simulink model "Cubesat_Control_PD"  (R2025b)
settings: Solver=ode45  StartTime=0.0  StopTime=t_stop  RelTol=1e-3
values from neighbouring files (symbols this model uses):
  J = 0.000634    [Matlab_to_BLE2.m]    (also in Run_CubeSat_HIL.m; init_simulation_lqr.m; init_simulation_pd.m)
  Jw = 4.607e-5    (= 4.607e-05)    [Matlab_to_BLE2.m]    (also in Run_CubeSat_HIL.m; init_simulation_lqr.m; init_simulation_pd.m)
  Kd = J * (3 * lambda - tau_delay)    [Matlab_to_BLE2.m]    (also in Run_CubeSat_HIL.m = 0.01; init_simulation_pd.m = J * (3 * lambda - tau))
  Kd_detumble = 0.03    [Matlab_to_BLE2.m]    (also in Run_CubeSat_HIL.m; init_simulation_lqr.m = lqr(A_d, B_d, Q_d, R_d); init_simulation_pd.m = 0.003)
  Ki = J * (lambda^3)    [Matlab_to_BLE2.m]    (also in init_simulation_pd.m)
  Kp = 3 * J * (lambda^2)    [Matlab_to_BLE2.m]    (also in Run_CubeSat_HIL.m = 0.02; init_simulation_pd.m)
  omega0 = deg2rad(omega0_deg)    [init_simulation_lqr.m]    (also in init_simulation_pd.m)
  omega_th_high = deg2rad(10)    [Run_CubeSat_HIL.m]    (also in init_simulation_lqr.m = deg2rad(10000); init_simulation_pd.m = deg2rad(10000))
  omega_th_low = deg2rad(2.0)    [Run_CubeSat_HIL.m]    (also in init_simulation_lqr.m = deg2rad(0.3); init_simulation_pd.m = deg2rad(0.3))
  omega_w0 = 0    [init_simulation_lqr.m]    (also in init_simulation_pd.m)
  tau = history_tau    [analyze_multiple_experiments.m]    (also in init_simulation_lqr.m = 2.3; init_simulation_pd.m = 2.3)
  tau_max = 0.2    [Matlab_to_BLE2.m]    (also in Run_CubeSat_HIL.m = 0.002; analyze_multiple_experiments.m = 0.002; init_simulation_lqr.m = 0.002; init_simulation_pd.m = 0.002)
  theta0 = theta(1)    [analyze_multiple_experiments.m]    (also in init_simulation_lqr.m = deg2rad(0); init_simulation_pd.m = deg2rad(0))
  theta_ref = deg2rad(theta_ref_deg)    [Matlab_to_BLE2.m]    (also in analyze_multiple_experiments.m = theta_ref_deg; init_simulation_lqr.m; init_simulation_pd.m)
settings Model: Creator=bbtp  LastModifiedBy=bbtp

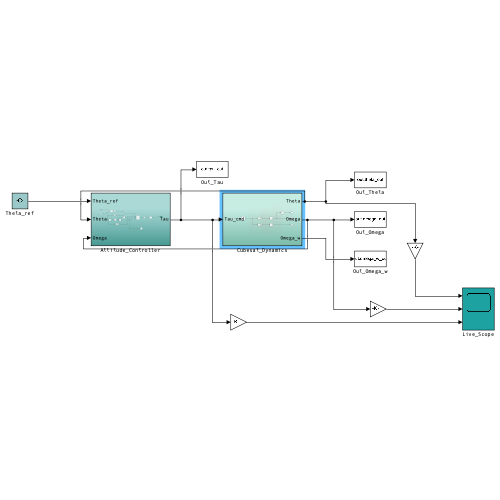
[thumbnail: Simulink's stored preview of the top-level diagram]
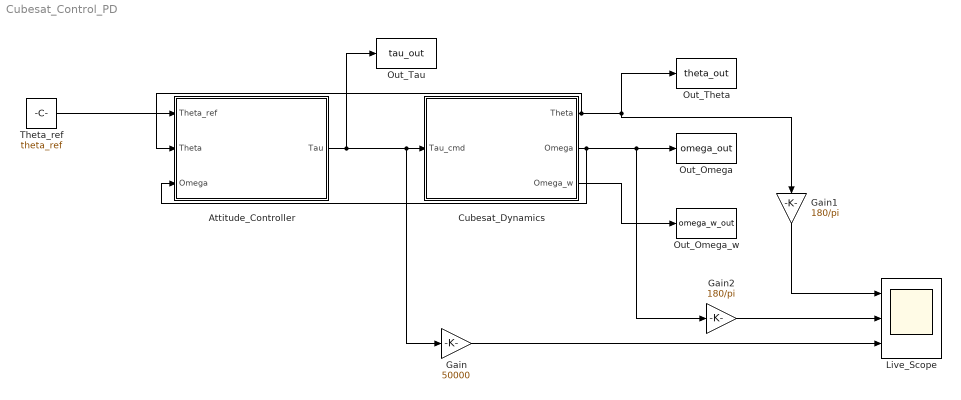
== system Cubesat_Control_PD ==
  Attitude_Controller : Subsystem
  Cubesat_Dynamics : Subsystem
  Gain : Gain  Gain=50000
  Gain1 : Gain  Gain=180/pi
  Gain2 : Gain  Gain=180/pi
  Live_Scope : Scope  NumInputPorts=3
      settings: ActiveDisplayYMinimum=-1  ActiveDisplayYMaximum=1
  Out_Omega : ToWorkspace  VariableName=omega_out  SampleTime=-1
  Out_Omega_w : ToWorkspace  VariableName=omega_w_out  SampleTime=-1
  Out_Tau : ToWorkspace  VariableName=tau_out  SampleTime=-1
  Out_Theta : ToWorkspace  VariableName=theta_out  SampleTime=-1
  Theta_ref : Constant  Value=theta_ref
  wires:
  Theta_ref/1 -> Attitude_Controller/1(Theta_ref)
  Attitude_Controller/1(Tau) -> Cubesat_Dynamics/1(Tau_cmd), Gain/1, Out_Tau/1
  Cubesat_Dynamics/1(Theta) -> Out_Theta/1, Gain1/1, Attitude_Controller/2(Theta)
  Cubesat_Dynamics/2(Omega) -> Out_Omega/1, Gain2/1, Attitude_Controller/3(Omega)
  Cubesat_Dynamics/3(Omega_w) -> Out_Omega_w/1
  Gain/1 -> Live_Scope/3
  Gain1/1 -> Live_Scope/1
  Gain2/1 -> Live_Scope/2

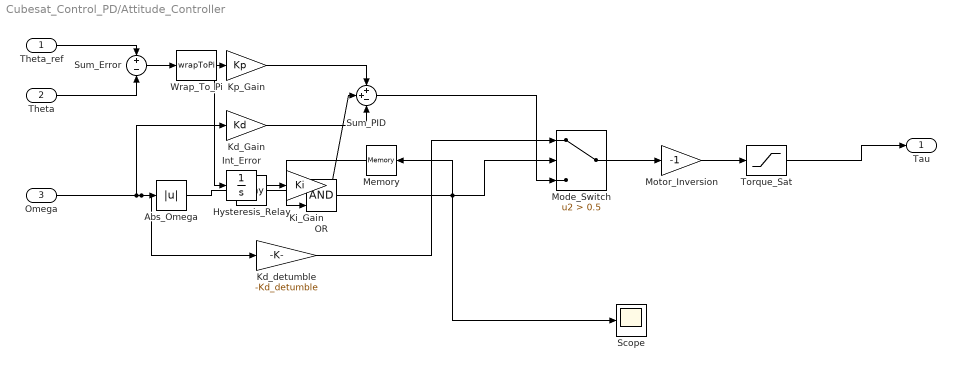
== system Cubesat_Control_PD/Attitude_Controller ==
  Theta_ref : Inport
  Theta : Inport  Port=2
  Omega : Inport  Port=3
  Abs_Omega : Abs  SaturateOnIntegerOverflow=off
  Hysteresis_Relay : Relay  OnSwitchValue=omega_th_high  OffSwitchValue=omega_th_low  InitialState=1
  Kd_Gain : Gain  Gain=Kd
  Kd_detumble : Gain  Gain=-Kd_detumble
  Kp_Gain : Gain  Gain=Kp
  Memory : Memory  InitialCondition=1
  Mode_Switch : Switch  Criteria=u2 > Threshold  Threshold=0.5  SaturateOnIntegerOverflow=off  InputSameDT=off
  Motor_Inversion : Gain  Gain=-1
  OR : Logic  IconShape=distinctive  AllPortsSameDT=off  OutDataTypeStr=boolean
  Scope : Scope
      settings: ActiveDisplayYMinimum=-1  ActiveDisplayYMaximum=1
  Sum_Error : Sum  Inputs=+-
  Sum_PID : Sum  Inputs=++-
  Int_Error : Integrator  InitialCondition=0
  Ki_Gain : Gain  Gain=Ki
  Torque_Sat : Saturate  UpperLimit=tau_max  LowerLimit=-tau_max
  Wrap_To_Pi : MATLABFcn  MATLABFcn=wrapToPi
  Tau : Outport
  wires:
  Theta_ref/1 -> Sum_Error/1
  Theta/1 -> Sum_Error/2
  Omega/1 -> Kd_detumble/1, Abs_Omega/1, Kd_Gain/1
  Kp_Gain/1 -> Sum_PID/1
  Kd_Gain/1 -> Sum_PID/3
  Int_Error/1 -> Ki_Gain/1
  Ki_Gain/1 -> Sum_PID/2
  Kd_detumble/1 -> Mode_Switch/1
  Abs_Omega/1 -> Hysteresis_Relay/1
  Sum_PID/1 -> Mode_Switch/3
  Mode_Switch/1 -> Motor_Inversion/1
  Motor_Inversion/1 -> Torque_Sat/1
  Torque_Sat/1 -> Tau/1
  Hysteresis_Relay/1 -> OR/1
  Memory/1 -> OR/2
  OR/1 -> Scope/1, Memory/1, Mode_Switch/2
  Sum_Error/1 -> Wrap_To_Pi/1
  Wrap_To_Pi/1 -> Kp_Gain/1, Int_Error/1

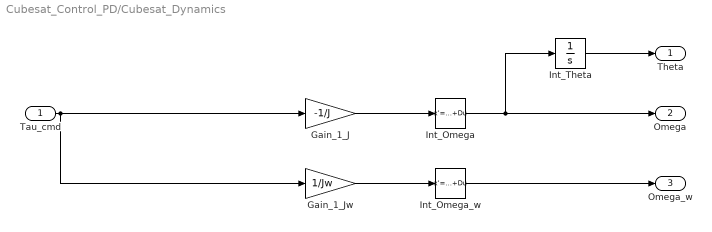
== system Cubesat_Control_PD/Cubesat_Dynamics ==
  Tau_cmd : Inport
  Gain_1_J : Gain  Gain=-1/J
  Gain_1_Jw : Gain  Gain=1/Jw
  Int_Omega : StateSpace  A=-tau  B=1  C=1  D=0  X0=omega0
  Int_Omega_w : StateSpace  A=-tau  B=1  C=1  D=0  X0=omega_w0
  Int_Theta : Integrator  InitialCondition=theta0
  Theta : Outport
  Omega : Outport  Port=2
  Omega_w : Outport  Port=3
  wires:
  Gain_1_Jw/1 -> Int_Omega_w/1
  Gain_1_J/1 -> Int_Omega/1
  Int_Omega/1 -> Int_Theta/1, Omega/1
  Int_Theta/1 -> Theta/1
  Int_Omega_w/1 -> Omega_w/1
  Tau_cmd/1 -> Gain_1_Jw/1, Gain_1_J/1
